simulink subsystem "check_conditions"  (R2024b)
settings: Solver=VariableStepAuto  StartTime=0.0  StopTime=10.0  RelTol=1e-3
undefined symbols (not defined in the file or in its folder): EnumPowerState
settings Model: Creator=developer  LastModifiedBy=developer

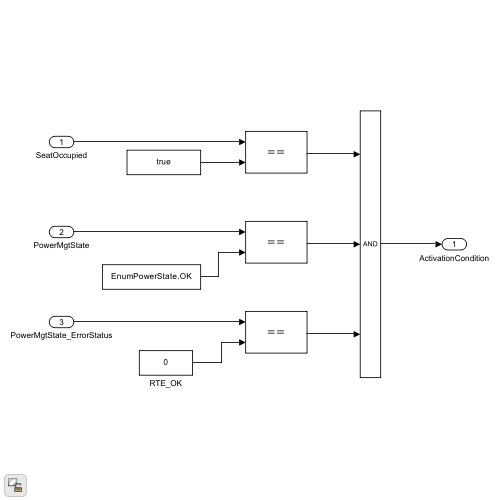
[thumbnail: Simulink's stored preview of the top-level diagram]
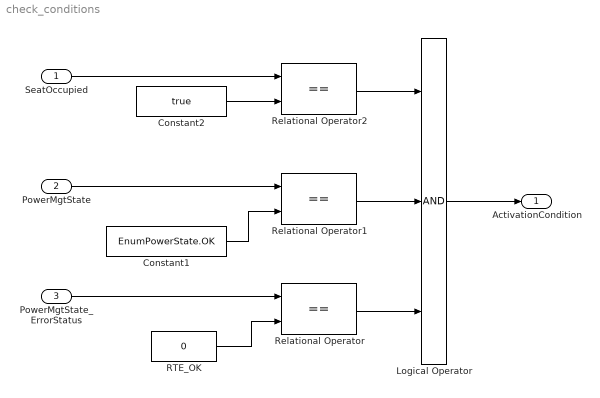
== system check_conditions ==
  SeatOccupied : Inport
  PowerMgtState : Inport  Port=2
  PowerMgtState_ErrorStatus : Inport  Port=3
  Constant1 : Constant  Value=EnumPowerState.OK
  Constant2 : Constant  Value=true
  Logical Operator : Logic  Inputs=3  AllPortsSameDT=off  OutDataTypeStr=boolean
  RTE_OK : Constant  Value=0
  Relational Operator : RelationalOperator  Operator===  OutDataTypeStr=boolean  RndMeth=Simplest  InputSameDT=off
  Relational Operator1 : RelationalOperator  Operator===  OutDataTypeStr=boolean  RndMeth=Simplest  InputSameDT=off
  Relational Operator2 : RelationalOperator  Operator===  OutDataTypeStr=boolean  RndMeth=Simplest  InputSameDT=off
  ActivationCondition : Outport  OutDataTypeStr=boolean  PortDimensions=1  InitialOutput=0
  wires:
  Logical Operator/1 -> ActivationCondition/1
  PowerMgtState_ErrorStatus/1 -> Relational Operator/1
  PowerMgtState/1 -> Relational Operator1/1
  Constant2/1 -> Relational Operator2/2
  SeatOccupied/1 -> Relational Operator2/1
  Relational Operator2/1 -> Logical Operator/1
  Constant1/1 -> Relational Operator1/2
  Relational Operator/1 -> Logical Operator/3
  Relational Operator1/1 -> Logical Operator/2
  RTE_OK/1 -> Relational Operator/2
